simulink model "single_phase_bridge_cr"  (Simulink 6.1)
settings: Solver=ode23tb  StartTime=0.0  StopTime=0.1499  MaxStep=1e-4  RelTol=1e-3  AbsTol=.01
libraries: powerlib x11
settings Model: LastModifiedBy=ThinkPad
settings DebuggingCC: SolverPrmCheckMsg=warning

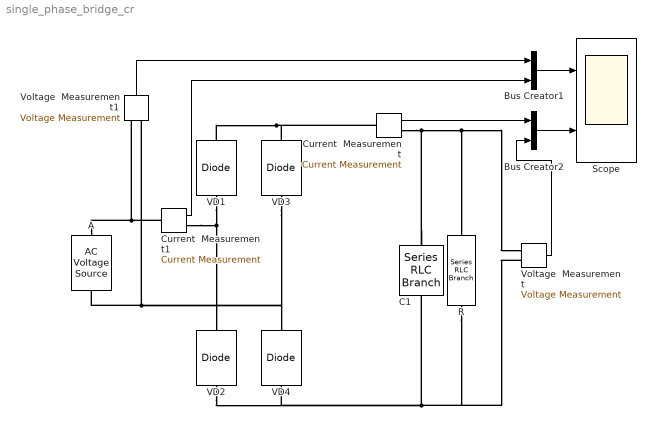
== system single_phase_bridge_cr ==
  A : powerlib/Electrical Sources/AC Voltage Source  Orientation=up  Amplitude=100  Phase=0  Frequency=50  SampleTime=0  Measurements=None
  Bus Creator1 : BusCreator  DialogController=Simulink.DDGSource_Bus  Inputs=2
  Bus Creator2 : BusCreator  DialogController=Simulink.DDGSource_Bus  Inputs=2
  C1 : powerlib/Elements/Series RLC Branch  Orientation=up  PhysicalDomain=powersysdomain  SubClassName=unknown  LeftPortType=p1  RightPortType=p1  LConnTagsString=__new0  RConnTagsString=__new0  Resistance=0  Inductance=0  Capacitance=0.001  Measurements=None
  Current  Measurement : powerlib/Measurements/Current Measurement  PhasorSimulation=off  OutputType=Complex  PSBequivalent=0
  Current  Measurement1 : powerlib/Measurements/Current Measurement  PhasorSimulation=off  OutputType=Complex  PSBequivalent=0
  R : powerlib/Elements/Series RLC Branch  Orientation=down  PhysicalDomain=powersysdomain  SubClassName=unknown  LeftPortType=p1  RightPortType=p1  LConnTagsString=__new0  RConnTagsString=__new0  Resistance=10  Inductance=0  Capacitance=inf  Measurements=None
  Scope : Scope  NumInputPorts=2
      settings: TimeRange=0.05  YMin=-100~0  YMax=100~100  Decimation=5  SampleInput=on  SampleTime=1e-4
  VD{1..4} (4 alike) : powerlib/Power Electronics/Diode  Orientation=up  Ron=0.001  Lon=0  Vf=0.8  IC=0  Rs=500  Cs=250e-9  Measurements=off
  Voltage  Measurement : powerlib/Measurements/Voltage Measurement  PhasorSimulation=off  OutputType=Complex  PSBequivalent=0
  Voltage  Measurement1 : powerlib/Measurements/Voltage Measurement  Orientation=up  PhasorSimulation=off  OutputType=Complex  PSBequivalent=0
  wires:
  Bus Creator1/1 -> Scope/1
  Voltage  Measurement1/1 -> Bus Creator1/1
  Current  Measurement1/1 -> Bus Creator1/2
  Current  Measurement/1 -> Bus Creator2/1
  Voltage  Measurement/1 -> Bus Creator2/2
  Bus Creator2/1 -> Scope/2
  connections:
  C1/RConn1 -- R/LConn1 -- Voltage  Measurement/LConn1 -- Current  Measurement/RConn1
  Current  Measurement/LConn1 -- VD1/RConn1 -- VD3/RConn1
  Current  Measurement1/LConn1 -- A/RConn1 -- Voltage  Measurement1/LConn1
  VD2/LConn1 -- VD4/LConn1 -- Voltage  Measurement/LConn2 -- R/RConn1 -- C1/LConn1
  VD3/LConn1 -- VD4/RConn1 -- A/LConn1 -- Voltage  Measurement1/LConn2
  VD1/LConn1 -- VD2/RConn1 -- Current  Measurement1/RConn1
